simulink model "lead_gradually_slows_down"  (R2025a)
settings: Solver=VariableStepAuto  StartTime=0.0  StopTime=20  RelTol=1e-3
settings Model: Creator=sanborkl  LastModifiedBy=admin

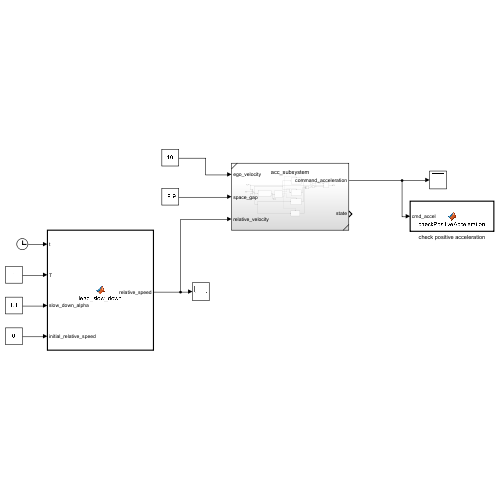
[thumbnail: Simulink's stored preview of the top-level diagram]
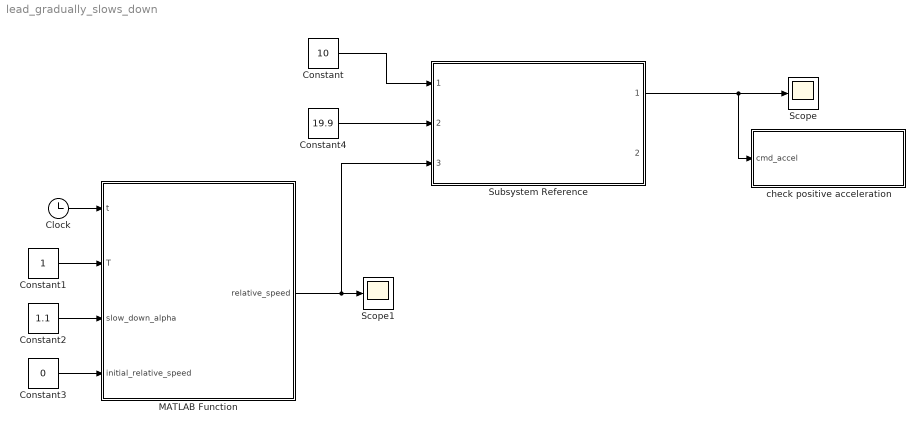
== system lead_gradually_slows_down ==
  Clock : Clock
  Constant : Constant  Value=10
  Constant1 : Constant
  Constant2 : Constant  Value=1.1
  Constant3 : Constant  Value=0
  Constant4 : Constant  Value=19.9
  MATLAB Function : MATLAB Function  TreatAsAtomicUnit=on
  Scope : Scope
      settings: ActiveDisplayYMinimum=-3.5828094546775495  ActiveDisplayYMaximum=1.322630956460404
  Scope1 : Scope
      settings: ActiveDisplayYMinimum=-1  ActiveDisplayYMaximum=1
  Subsystem Reference : Subsystem  ReferencedSubsystem=acc_subsystem
  check positive acceleration : MATLAB Function  TreatAsAtomicUnit=on
  wires:
  Constant/1 -> Subsystem Reference/1
  Clock/1 -> MATLAB Function/1(t)
  Subsystem Reference/1 -> check positive acceleration/1(cmd_accel), Scope/1
  Constant1/1 -> MATLAB Function/2(T)
  Constant2/1 -> MATLAB Function/3(slow_down_alpha)
  Constant3/1 -> MATLAB Function/4(initial_relative_speed)
  MATLAB Function/1(relative_speed) -> Subsystem Reference/3, Scope1/1
  Constant4/1 -> Subsystem Reference/2

== matlab function lead_gradually_slows_down/MATLAB Function ==
  data: t input; relative_speed output; T input; slow_down_alpha input; initial_relative_speed input
function relative_speed = lead_slow_down(t, T, slow_down_alpha, initial_relative_speed)

if (t < T)
    relative_speed = initial_relative_speed;
else
    relative_speed = initial_relative_speed + -(slow_down_alpha * t);
end

== matlab function lead_gradually_slows_down/check positive acceleration ==
  data: cmd_accel input
function checkPositiveAcceleration(cmd_accel)
%#codegen
coder.extrinsic('disp', 'sprintf');

if cmd_accel < 0
    msg = sprintf('Error: Negative command acceleration: %.3f, should be positive', ...
                  cmd_accel);
    disp(msg);
end
end
